simulink library "lib_BMS_2019b"  (R2020a)
settings: Solver=VariableStepAuto  StartTime=0.0  StopTime=10.0  RelTol=1e-3
undefined symbols (not defined in the file): OCVdata
libraries: simulink x4
settings Model: Creator=wzhao  LastModifiedBy="wei  zhao"
settings DebuggingCC: ArithmeticOperatorsInVariantConditions=warning
settings SFSimCC: CustomCodeUndefinedFunction=UseInterfaceOnly
settings RTWCC: GenCodeOnly=on

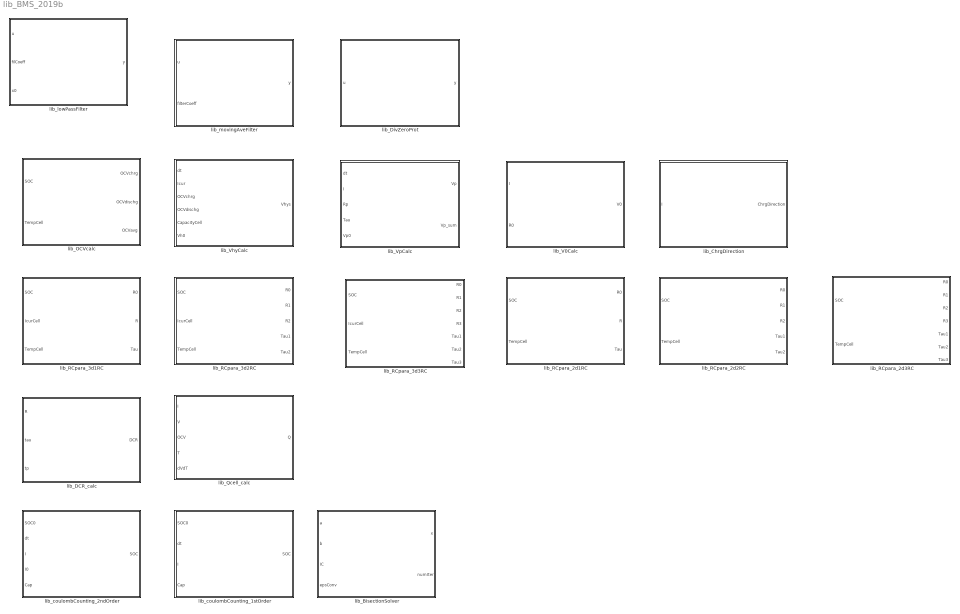
== system lib_BMS_2019b ==
  lib_BisectionSolver : Subsystem  TreatAsAtomicUnit=on  mask{myAlias_parameter=0, iterMax=10}
      mask prompts: myAlias_parameter "fx function data type"; iterMax "Maximum Iteration Number"
  lib_ChrgDirection : Subsystem  mask{ChrgFlag=0, DischrgFlag=0, Imin=0}
      mask prompts: ChrgFlag "Charge flag"; DischrgFlag "Discharge flag"; Imin "Min Current Tolerance"
  lib_DCR_calc : Subsystem  TreatAsAtomicUnit=on
  lib_DivZeroProt : Subsystem  TreatAsAtomicUnit=on  mask{epsilon=0, Default_value=0}
      mask prompts: epsilon "Divde-by-zero tolerance"; Default_value "Default Value"
  lib_OCVcalc : Subsystem  mask{OCVdata=OCVdata}
      mask prompts: OCVdata "OCV data."
  lib_Qcell_calc : Subsystem  TreatAsAtomicUnit=on
  lib_RCpara_2d1RC : Subsystem  TreatAsAtomicUnit=on  mask{xTemp=[1 2], xsoc=[1 2], yR0=zeros(2,2), yR=zeros(2,2), yTau=zeros(2,2)}
      mask prompts: xTemp "Temperature breakpoints"; xsoc "SOC breakpoints"; yR0 "R0 data"; yR "R data"; yTau "Tau data"
      mask DialogControl Container7 Prompt: Breakpoints
      mask DialogControl Container9 Prompt: RC data
  lib_RCpara_2d2RC : Subsystem  TreatAsAtomicUnit=on  mask{xTemp=[1 2], xsoc=[1 2], yR0=zeros(2,2), yR1=zeros(2,2), yR2=zeros(2,2), yTau1=zeros(2,2), yTau2=zeros(2,2)}
      mask prompts: xTemp "Temperature breakpoints"; xsoc "SOC breakpoints"; yR0 "R0 data"; yR1 "R1 data"; yR2 "R2 data"; yTau1 "Tau1 data"; yTau2 "Tau2 data"
      mask DialogControl Container7 Prompt: Breakpoints
      mask DialogControl Container9 Prompt: RC data
  lib_RCpara_2d3RC : Subsystem  TreatAsAtomicUnit=on  mask{xTemp=[1 2], xsoc=[1 2], yR0=zeros(2,2), yR1=zeros(2,2), yR2=zeros(2,2), yR3=zeros(2,2), yTau1=zeros(2,2), yTau2=zeros(2,2), yTau3=zeros(2,2)}
      mask prompts: xTemp "Temperature breakpoints"; xsoc "SOC breakpoints"; yR0 "R0 data"; yR1 "R1 data"; yR2 "R2 data"; yR3 "R3 data"; yTau1 "Tau1 data"; yTau2 "Tau2 data"; yTau3 "Tau3 data"
      mask DialogControl Container7 Prompt: Breakpoints
      mask DialogControl Container9 Prompt: RC data
  lib_RCpara_3d1RC : Subsystem  TreatAsAtomicUnit=on  mask{xsoc=[1 2], xIcurCell=[1 2], xTemp=[1 2], yR0=0, yR=zeros(2,2,2), yTau=zeros(2,2,2)}
      mask prompts: xsoc "SOC breakpoints"; xIcurCell "Current breakpoints"; xTemp "Temperature breakpoints"; yR0 "R0 data"; yR "R data"; yTau "Tau data"
      mask DialogControl Container7 Prompt: Breakpoints
      mask DialogControl Container10 Prompt: Tab
      mask DialogControl Container9 Prompt: RC data
  lib_RCpara_3d2RC : Subsystem  TreatAsAtomicUnit=on  mask{xsoc=[1 2], xIcurCell=[1 2], xTemp=[1 2], yR0=zeros(2,2,2), yR1=zeros(2,2,2), yR2=zeros(2,2,2), yTau1=zeros(2,2,2), yTau2=zeros(2,2,2)}
      mask prompts: xsoc "SOC breakpoints"; xIcurCell "Current breakpoints"; xTemp "Temperature breakpoints"; yR0 "R0 data"; yR1 "R1 data"; yR2 "R2 data"; yTau1 "Tau1 data"; yTau2 "Tau2 data"
      mask DialogControl Container7 Prompt: Breakpoints
      mask DialogControl Container9 Prompt: RC data
  lib_RCpara_3d3RC : Subsystem  TreatAsAtomicUnit=on  mask{xsoc=[1 2], xIcurCell=[1 2], xTemp=[1 2], yR0=zeros(2,2,2), yR1=zeros(2,2,2), yR2=zeros(2,2,2), yR3=zeros(2,2,2), yTau1=zeros(2,2,2), yTau2=zeros(2,2,2), yTau3=zeros(2,2,2)}
      mask prompts: xsoc "SOC breakpoints"; xIcurCell "Current breakpoints"; xTemp "Temperature breakpoints"; yR0 "R0 data"; yR1 "R1 data"; yR2 "R2 data"; yR3 "R3 data"; yTau1 "Tau1 data"; yTau2 "Tau2 data"; yTau3 "Tau3 data"
      mask DialogControl Container7 Prompt: Breakpoints
      mask DialogControl Container9 Prompt: RC data
  lib_V0Calc : Subsystem  TreatAsAtomicUnit=on
  lib_VhyCalc : Subsystem  mask{Isign=1, Vh_para=0}
      mask prompts: Isign "Current Sign Convention(+is charge, - is negative)"; Vh_para "Vh parameter"
  lib_VpCalc : Subsystem  TreatAsAtomicUnit=on
  lib_coulombCounting_1stOrder : Subsystem  mask{Isign=0, unitConv=0}
      mask prompts: Isign "Discharge Current Sign"; unitConv "Unit Conversion Factor"
  lib_coulombCounting_2ndOrder : Subsystem  mask{Isign=0, unitConv=0}
      mask prompts: Isign "Charge Current Sign"; unitConv "Unit Conversion factor"
  lib_lowPassFilter : Subsystem  TreatAsAtomicUnit=on  RTWFcnName=lib_lowPassFilter
  lib_movingAveFilter : Subsystem  TreatAsAtomicUnit=on  mask{x0=0}
      mask prompts: x0 "Initial filter states"

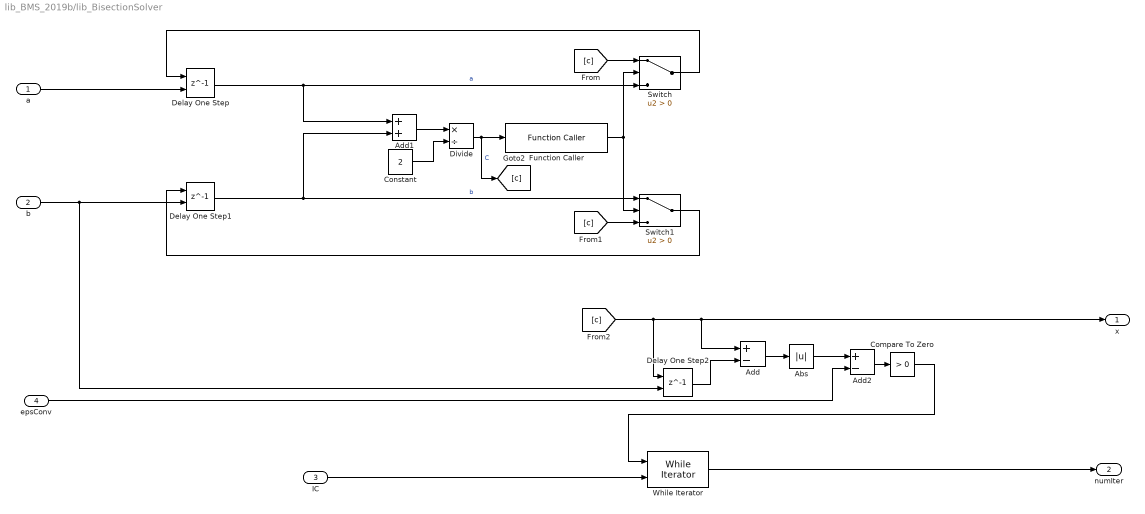
== system lib_BMS_2019b/lib_BisectionSolver ==
  a : Inport
  b : Inport  Port=2
  IC : Inport  Port=3
  epsConv : Inport  Port=4
  Abs : Abs
  Add : Sum  Inputs=+-
  Add1 : Sum
  Add2 : Sum  Inputs=+-
  Compare To Zero : simulink/Logic and Bit Operations/Compare To Zero  relop=>  OutDataTypeStr=boolean
  Constant : Constant  Value=2  OutDataTypeStr=Inherit: Inherit via back propagation  SampleTime=-1
  Delay One Step : Delay  DelayLength=1  InitialConditionSource=Input port
      settings: InputPortMap=u0,p4
  Delay One Step1 : Delay  DelayLength=1  InitialConditionSource=Input port
      settings: InputPortMap=u0,p4
  Delay One Step2 : Delay  DelayLength=1  InitialConditionSource=Input port
      settings: InputPortMap=u0,p4
  Divide : Product  Inputs=*/
  Function Caller : FunctionCaller  FunctionPrototype=y = funcToSolveBisec(u)  InputArgumentSpecifications=myAlias_parameter  OutputArgumentSpecifications=myAlias_parameter
  Switch : Switch  Criteria=u2 > Threshold
  Switch1 : Switch  Criteria=u2 > Threshold
  While Iterator : WhileIterator  MaxIters=iterMax  ResetStates=reset  ShowIterationPort=on
  x : Outport
  numIter : Outport  Port=2
  wires:
  IC/1 -> While Iterator/2
  [c] -> Add/1, x/1, Delay One Step2/1
  Delay One Step2/1 -> Add/2
  Add/1 -> Abs/1
  Abs/1 -> Add2/1
  Compare To Zero/1 -> While Iterator/1
  a/1 -> Delay One Step/2
  b/1 -> Delay One Step2/2, Delay One Step1/2
  Delay One Step/1 -> Add1/1, Switch/3  "a"
  Delay One Step1/1 -> Add1/2, Switch1/1  "b"
  Add1/1 -> Divide/1
  Constant/1 -> Divide/2
  Divide/1 -> [c], Function Caller/1  "C"
  Function Caller/1 -> Switch1/2, Switch/2
  [c] -> Switch/1
  [c] -> Switch1/3
  Switch/1 -> Delay One Step/1
  Switch1/1 -> Delay One Step1/1
  epsConv/1 -> Add2/2
  Add2/1 -> Compare To Zero/1
  While Iterator/1 -> numIter/1

== system lib_BMS_2019b/lib_ChrgDirection ==
  I : Inport
  Compare To Constant : simulink/Logic and Bit Operations/Compare To Constant  relop=>=  const=Imin  OutDataTypeStr=boolean
  Compare To Constant1 : simulink/Logic and Bit Operations/Compare To Constant  relop=<=  const=-Imin  OutDataTypeStr=boolean
  Constant : Constant  Value=ChrgFlag
  Constant1 : Constant  Value=DischrgFlag
  Switch : Switch  Criteria=u2 ~= 0
  Switch1 : Switch  Criteria=u2 ~= 0
  Unit Delay : UnitDelay  InitialCondition=ChrgFlag  SampleTime=-1  HasFrameUpgradeWarning=on
  ChrgDirection : Outport
  wires:
  I/1 -> Compare To Constant1/1, Compare To Constant/1
  Compare To Constant/1 -> Switch/2
  Constant/1 -> Switch/1
  Compare To Constant1/1 -> Switch1/2
  Switch1/1 -> Switch/3
  Constant1/1 -> Switch1/1
  Switch/1 -> ChrgDirection/1, Unit Delay/1
  Unit Delay/1 -> Switch1/3

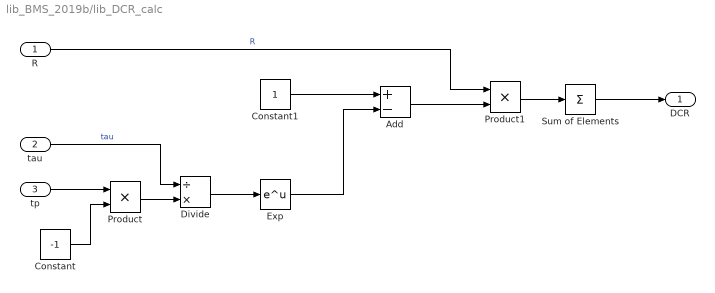
== system lib_BMS_2019b/lib_DCR_calc ==
  R : Inport
  tau : Inport  Port=2
  tp : Inport  Port=3
  Add : Sum  Inputs=+-
  Constant : Constant  Value=-1  OutDataTypeStr=Inherit: Inherit via back propagation
  Constant1 : Constant  OutDataTypeStr=Inherit: Inherit via back propagation
  Divide : Product  Inputs=/*
  Exp : Math  SaturateOnIntegerOverflow=on
  Product : Product
  Product1 : Product
  Sum of Elements : Sum  Inputs=+
  DCR : Outport
  wires:
  Sum of Elements/1 -> DCR/1
  tp/1 -> Product/1
  Constant/1 -> Product/2
  Product/1 -> Divide/2
  tau/1 -> Divide/1  "tau"
  Divide/1 -> Exp/1
  Exp/1 -> Add/2
  Product1/1 -> Sum of Elements/1
  Constant1/1 -> Add/1
  Add/1 -> Product1/2
  R/1 -> Product1/1  "R"

== system lib_BMS_2019b/lib_DivZeroProt ==
  u : Inport
  Abs : Abs
  Compare To Constant : simulink/Logic and Bit Operations/Compare To Constant  relop=<=  const=epsilon  OutDataTypeStr=boolean
  Constant2 : Constant  Value=Default_value
  Switch : Switch  Criteria=u2 ~= 0
  y : Outport
  wires:
  Constant2/1 -> Switch/1
  Compare To Constant/1 -> Switch/2
  u/1 -> Switch/3, Abs/1
  Abs/1 -> Compare To Constant/1
  Switch/1 -> y/1

== system lib_BMS_2019b/lib_OCVcalc ==
  SOC : Inport
  TempCell : Inport  Port=2
  1-D Lookup Table : Lookup_n-D  BreakpointsForDimension1=OCVdata.xSOC  BreakpointsForDimension2=OCVdata.xTemp  Table=OCVdata.yOCVc  InternalRulePriority=Speed  RndMeth=Simplest  InputSameDT=on
  1-D Lookup Table1 : Lookup_n-D  BreakpointsForDimension1=OCVdata.xSOC  BreakpointsForDimension2=OCVdata.xTemp  Table=OCVdata.yOCVd  InternalRulePriority=Speed  RndMeth=Simplest  InputSameDT=on
  Add : Sum
  Constant : Constant  Value=2  OutDataTypeStr=Inherit: Inherit via back propagation
  Divide : Product  Inputs=*/
  OCVchrg : Outport
  OCVdischg : Outport  Port=2
  OCVavg : Outport  Port=3
  wires:
  SOC/1 -> 1-D Lookup Table1/1, 1-D Lookup Table/1
  TempCell/1 -> 1-D Lookup Table1/2, 1-D Lookup Table/2
  1-D Lookup Table/1 -> Add/1, OCVchrg/1
  1-D Lookup Table1/1 -> OCVdischg/1, Add/2
  Add/1 -> Divide/1
  Constant/1 -> Divide/2
  Divide/1 -> OCVavg/1

== system lib_BMS_2019b/lib_Qcell_calc ==
  I : Inport
  V : Inport  Port=2
  OCV : Inport  Port=3
  T : Inport  Port=4
  dVdT : Inport  Port=5
  Abs : Abs
  Add : Sum  Inputs=-+
  Add1 : Sum
  Product : Product
  Product1 : Product  Inputs=3
  Q : Outport
  wires:
  V/1 -> Add/1
  OCV/1 -> Add/2
  Add/1 -> Product/2
  I/1 -> Product1/1, Product/1
  Product/1 -> Abs/1
  T/1 -> Product1/2
  dVdT/1 -> Product1/3
  Abs/1 -> Add1/1  "Qire"
  Product1/1 -> Add1/2  "Qrev"
  Add1/1 -> Q/1

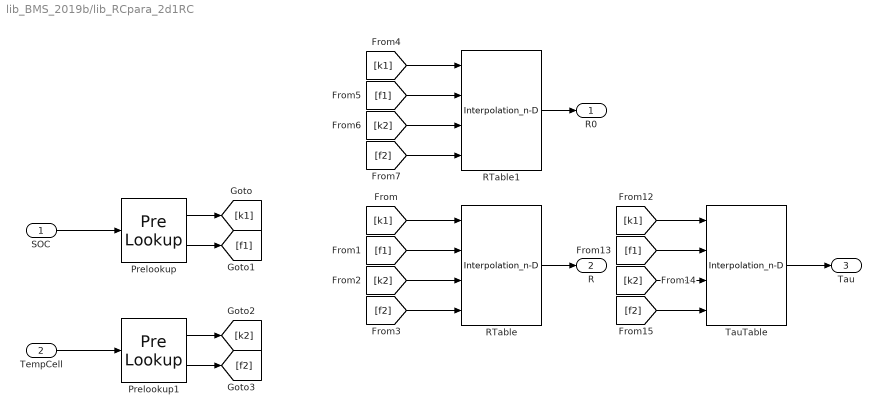
== system lib_BMS_2019b/lib_RCpara_2d1RC ==
  SOC : Inport
  TempCell : Inport  Port=2
  Prelookup : PreLookup  BreakpointsData=xsoc  ExtrapMethod=Linear
  Prelookup1 : PreLookup  BreakpointsData=xTemp  ExtrapMethod=Linear
  RTable : Interpolation_n-D  Table=yR  InternalRulePriority=Speed
  RTable1 : Interpolation_n-D  Table=yR0  InternalRulePriority=Speed
  TauTable : Interpolation_n-D  Table=yTau  InternalRulePriority=Speed
  R0 : Outport
  R : Outport  Port=2
  Tau : Outport  Port=3
  wires:
  Prelookup1/2 -> [f2]
  [k1] -> TauTable/1
  [f2] -> TauTable/4
  Prelookup/2 -> [f1]
  TauTable/1 -> Tau/1
  [k2] -> RTable/3
  [f2] -> RTable/4
  [k2] -> TauTable/3
  [f1] -> TauTable/2
  TempCell/1 -> Prelookup1/1
  Prelookup/1 -> [k1]
  [k1] -> RTable/1
  SOC/1 -> Prelookup/1
  Prelookup1/1 -> [k2]
  RTable/1 -> R/1
  [f1] -> RTable/2
  [f2] -> RTable1/4
  [f1] -> RTable1/2
  [k2] -> RTable1/3
  [k1] -> RTable1/1
  RTable1/1 -> R0/1

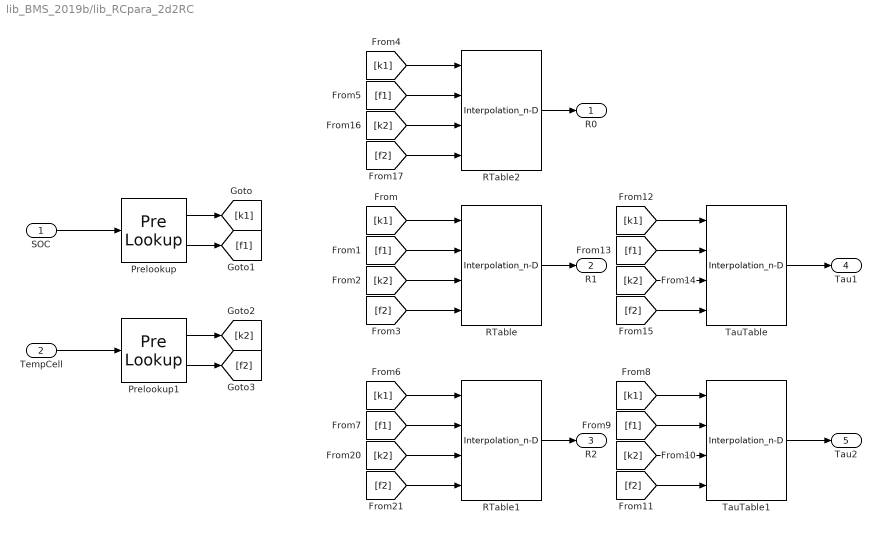
== system lib_BMS_2019b/lib_RCpara_2d2RC ==
  SOC : Inport
  TempCell : Inport  Port=2
  Prelookup : PreLookup  BreakpointsData=xsoc  ExtrapMethod=Linear
  Prelookup1 : PreLookup  BreakpointsData=xTemp  ExtrapMethod=Linear
  RTable : Interpolation_n-D  Table=yR1  InternalRulePriority=Speed
  RTable1 : Interpolation_n-D  Table=yR2  InternalRulePriority=Speed
  RTable2 : Interpolation_n-D  Table=yR0  InternalRulePriority=Speed
  TauTable : Interpolation_n-D  Table=yTau1  InternalRulePriority=Speed
  TauTable1 : Interpolation_n-D  Table=yTau2  InternalRulePriority=Speed
  R0 : Outport
  R1 : Outport  Port=2
  R2 : Outport  Port=3
  Tau1 : Outport  Port=4
  Tau2 : Outport  Port=5
  wires:
  Prelookup1/2 -> [f2]
  [k1] -> TauTable/1
  [f2] -> TauTable/4
  Prelookup/2 -> [f1]
  TauTable/1 -> Tau1/1
  [k2] -> RTable/3
  [f2] -> RTable/4
  [k2] -> TauTable/3
  [f1] -> TauTable/2
  TempCell/1 -> Prelookup1/1
  Prelookup/1 -> [k1]
  [k1] -> RTable/1
  SOC/1 -> Prelookup/1
  Prelookup1/1 -> [k2]
  RTable/1 -> R1/1
  [f1] -> RTable/2
  [f1] -> RTable1/2
  [k1] -> RTable1/1
  RTable1/1 -> R2/1
  [f2] -> RTable1/4
  [k2] -> TauTable1/3
  TauTable1/1 -> Tau2/1
  [k2] -> RTable1/3
  [f1] -> TauTable1/2
  [k1] -> TauTable1/1
  [f2] -> TauTable1/4
  [k1] -> RTable2/1
  [f1] -> RTable2/2
  [k2] -> RTable2/3
  [f2] -> RTable2/4
  RTable2/1 -> R0/1

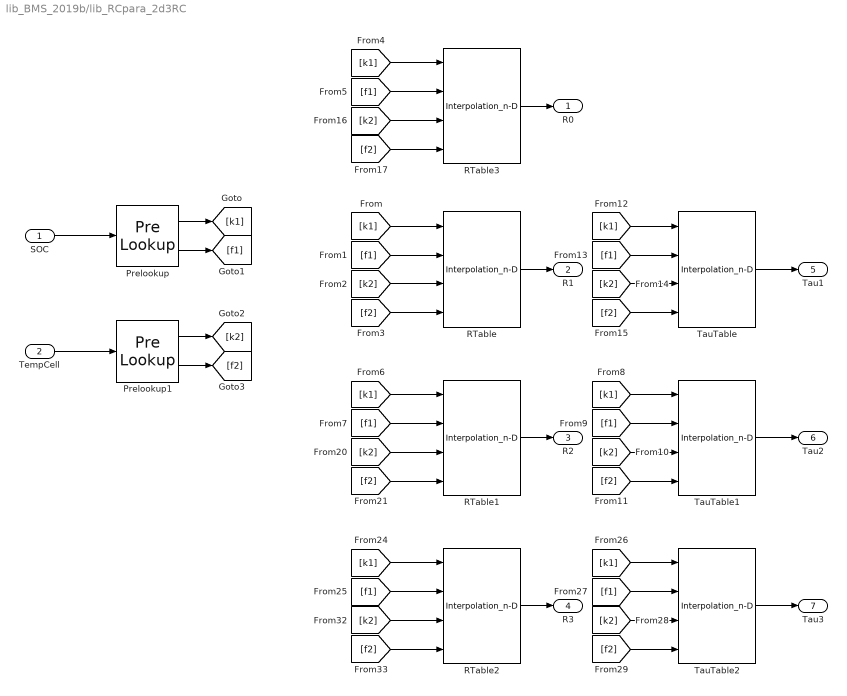
== system lib_BMS_2019b/lib_RCpara_2d3RC ==
  SOC : Inport
  TempCell : Inport  Port=2
  Prelookup : PreLookup  BreakpointsData=xsoc  ExtrapMethod=Linear
  Prelookup1 : PreLookup  BreakpointsData=xTemp  ExtrapMethod=Linear
  RTable : Interpolation_n-D  Table=yR1  InternalRulePriority=Speed
  RTable1 : Interpolation_n-D  Table=yR2  InternalRulePriority=Speed
  RTable2 : Interpolation_n-D  Table=yR3  InternalRulePriority=Speed
  RTable3 : Interpolation_n-D  Table=yR0  InternalRulePriority=Speed
  TauTable : Interpolation_n-D  Table=yTau1  InternalRulePriority=Speed
  TauTable1 : Interpolation_n-D  Table=yTau2  InternalRulePriority=Speed
  TauTable2 : Interpolation_n-D  Table=yTau3  InternalRulePriority=Speed
  R0 : Outport
  R1 : Outport  Port=2
  R2 : Outport  Port=3
  R3 : Outport  Port=4
  Tau1 : Outport  Port=5
  Tau2 : Outport  Port=6
  Tau3 : Outport  Port=7
  wires:
  Prelookup1/2 -> [f2]
  [k1] -> TauTable/1
  [f2] -> TauTable/4
  Prelookup/2 -> [f1]
  TauTable/1 -> Tau1/1
  [k2] -> RTable/3
  [f2] -> RTable/4
  [k2] -> TauTable/3
  [f1] -> TauTable/2
  TempCell/1 -> Prelookup1/1
  Prelookup/1 -> [k1]
  [k1] -> RTable/1
  SOC/1 -> Prelookup/1
  Prelookup1/1 -> [k2]
  RTable/1 -> R1/1
  [f1] -> RTable/2
  [f1] -> RTable1/2
  [k1] -> RTable1/1
  RTable1/1 -> R2/1
  [f2] -> RTable1/4
  [k2] -> TauTable1/3
  TauTable1/1 -> Tau2/1
  [k2] -> RTable1/3
  [f1] -> TauTable1/2
  [k1] -> TauTable1/1
  [f2] -> TauTable1/4
  [f1] -> RTable2/2
  [k1] -> RTable2/1
  RTable2/1 -> R3/1
  [f2] -> RTable2/4
  [k2] -> TauTable2/3
  TauTable2/1 -> Tau3/1
  [k2] -> RTable2/3
  [f1] -> TauTable2/2
  [k1] -> TauTable2/1
  [f2] -> TauTable2/4
  [f2] -> RTable3/4
  RTable3/1 -> R0/1
  [k1] -> RTable3/1
  [k2] -> RTable3/3
  [f1] -> RTable3/2

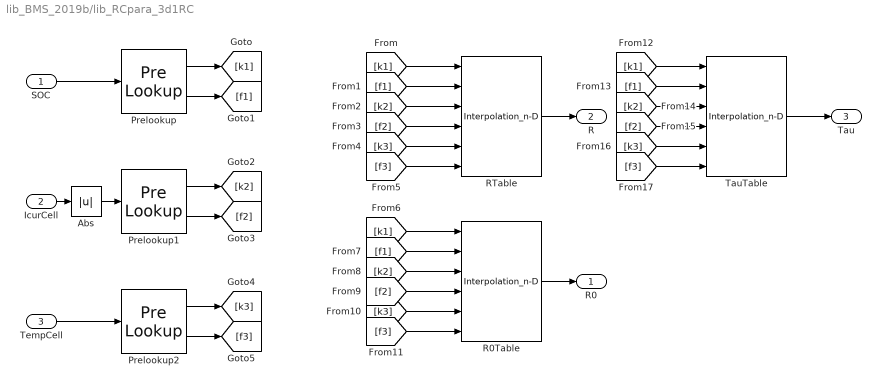
== system lib_BMS_2019b/lib_RCpara_3d1RC ==
  SOC : Inport
  IcurCell : Inport  Port=2
  TempCell : Inport  Port=3
  Abs : Abs
  Prelookup : PreLookup  BreakpointsData=xsoc  ExtrapMethod=Linear
  Prelookup1 : PreLookup  BreakpointsData=xIcurCell  ExtrapMethod=Linear
  Prelookup2 : PreLookup  BreakpointsData=xTemp  ExtrapMethod=Linear
  R0Table : Interpolation_n-D  NumberOfTableDimensions=3  Table=yR0  InternalRulePriority=Speed
      settings: InputPortMap=u0,u1,u2,u3,u4,u5
  RTable : Interpolation_n-D  NumberOfTableDimensions=3  Table=yR  InternalRulePriority=Speed
      settings: InputPortMap=u0,u1,u2,u3,u4,u5
  TauTable : Interpolation_n-D  NumberOfTableDimensions=3  Table=yTau  InternalRulePriority=Speed
      settings: InputPortMap=u0,u1,u2,u3,u4,u5
  R0 : Outport
  R : Outport  Port=2
  Tau : Outport  Port=3
  wires:
  Prelookup1/2 -> [f2]
  [k1] -> TauTable/1
  [f2] -> TauTable/4
  [k3] -> RTable/5
  Prelookup/2 -> [f1]
  TauTable/1 -> Tau/1
  [k2] -> RTable/3
  [f3] -> RTable/6
  [f2] -> RTable/4
  [f3] -> TauTable/6
  [k2] -> TauTable/3
  [k3] -> TauTable/5
  [f1] -> TauTable/2
  Prelookup/1 -> [k1]
  [k1] -> RTable/1
  SOC/1 -> Prelookup/1
  TempCell/1 -> Prelookup2/1
  Prelookup2/2 -> [f3]
  Prelookup2/1 -> [k3]
  Prelookup1/1 -> [k2]
  RTable/1 -> R/1
  [f1] -> RTable/2
  [k2] -> R0Table/3
  [f3] -> R0Table/6
  [k1] -> R0Table/1
  [f2] -> R0Table/4
  R0Table/1 -> R0/1
  [f1] -> R0Table/2
  [k3] -> R0Table/5
  IcurCell/1 -> Abs/1
  Abs/1 -> Prelookup1/1

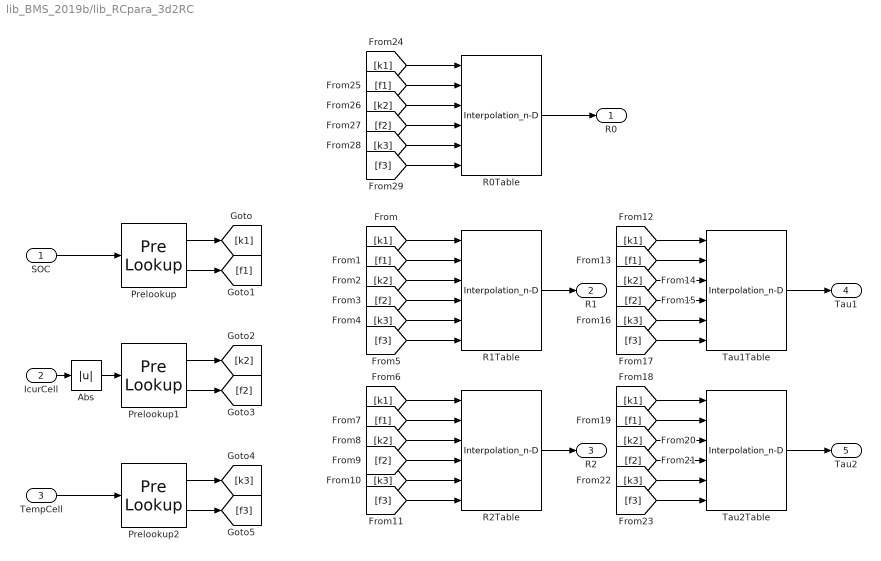
== system lib_BMS_2019b/lib_RCpara_3d2RC ==
  SOC : Inport
  IcurCell : Inport  Port=2
  TempCell : Inport  Port=3
  Abs : Abs
  Prelookup : PreLookup  BreakpointsData=xsoc  ExtrapMethod=Linear
  Prelookup1 : PreLookup  BreakpointsData=xIcurCell  ExtrapMethod=Linear
  Prelookup2 : PreLookup  BreakpointsData=xTemp  ExtrapMethod=Linear
  R0Table : Interpolation_n-D  NumberOfTableDimensions=3  Table=yR0  InternalRulePriority=Speed
      settings: InputPortMap=u0,u1,u2,u3,u4,u5
  R1Table : Interpolation_n-D  NumberOfTableDimensions=3  Table=yR1  InternalRulePriority=Speed
      settings: InputPortMap=u0,u1,u2,u3,u4,u5
  R2Table : Interpolation_n-D  NumberOfTableDimensions=3  Table=yR2  InternalRulePriority=Speed
      settings: InputPortMap=u0,u1,u2,u3,u4,u5
  Tau1Table : Interpolation_n-D  NumberOfTableDimensions=3  Table=yTau1  InternalRulePriority=Speed
      settings: InputPortMap=u0,u1,u2,u3,u4,u5
  Tau2Table : Interpolation_n-D  NumberOfTableDimensions=3  Table=yTau2  InternalRulePriority=Speed
      settings: InputPortMap=u0,u1,u2,u3,u4,u5
  R0 : Outport
  R1 : Outport  Port=2
  R2 : Outport  Port=3
  Tau1 : Outport  Port=4
  Tau2 : Outport  Port=5
  wires:
  Prelookup1/2 -> [f2]
  [k3] -> Tau2Table/5
  [k1] -> Tau1Table/1
  [f2] -> Tau1Table/4
  [k3] -> R1Table/5
  [f2] -> R2Table/4
  Prelookup/2 -> [f1]
  Tau1Table/1 -> Tau1/1
  [k2] -> R1Table/3
  [k1] -> R2Table/1
  [k1] -> Tau2Table/1
  [f3] -> R1Table/6
  R2Table/1 -> R2/1
  [f2] -> R1Table/4
  [f1] -> Tau2Table/2
  [f3] -> Tau1Table/6
  [k2] -> Tau1Table/3
  [k3] -> Tau1Table/5
  [f1] -> Tau1Table/2
  [k2] -> Tau2Table/3
  [f3] -> Tau2Table/6
  [f2] -> Tau2Table/4
  Prelookup/1 -> [k1]
  [k1] -> R1Table/1
  Tau2Table/1 -> Tau2/1
  SOC/1 -> Prelookup/1
  TempCell/1 -> Prelookup2/1
  Prelookup2/2 -> [f3]
  Prelookup2/1 -> [k3]
  Prelookup1/1 -> [k2]
  R1Table/1 -> R1/1
  [k3] -> R2Table/5
  [f1] -> R2Table/2
  [f1] -> R1Table/2
  [f3] -> R2Table/6
  [k2] -> R2Table/3
  [k2] -> R0Table/3
  [f3] -> R0Table/6
  [k3] -> R0Table/5
  [k1] -> R0Table/1
  [f1] -> R0Table/2
  [f2] -> R0Table/4
  R0Table/1 -> R0/1
  IcurCell/1 -> Abs/1
  Abs/1 -> Prelookup1/1

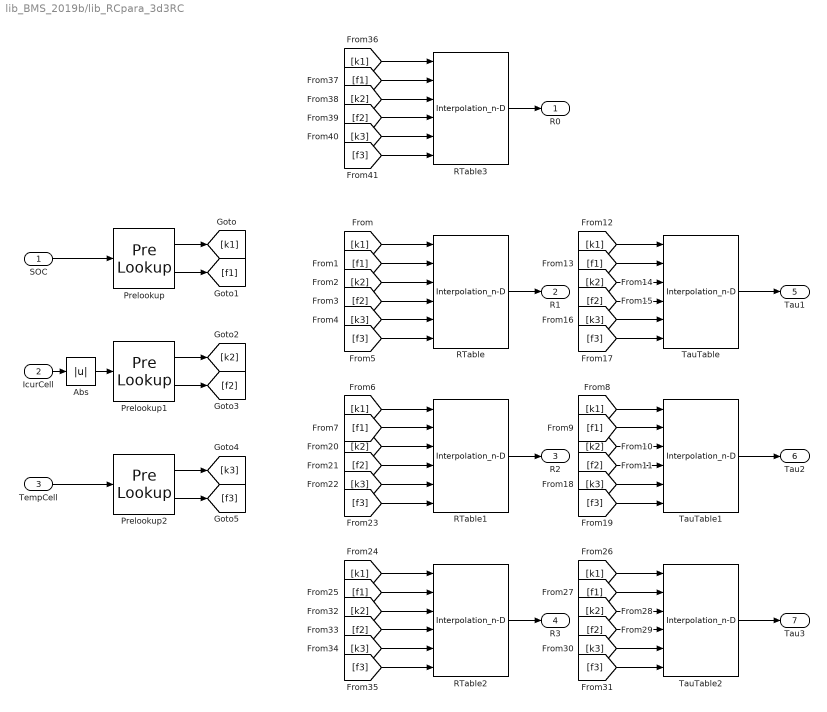
== system lib_BMS_2019b/lib_RCpara_3d3RC ==
  SOC : Inport
  IcurCell : Inport  Port=2
  TempCell : Inport  Port=3
  Abs : Abs
  Prelookup : PreLookup  BreakpointsData=xsoc  ExtrapMethod=Linear
  Prelookup1 : PreLookup  BreakpointsData=xIcurCell  ExtrapMethod=Linear
  Prelookup2 : PreLookup  BreakpointsData=xTemp  ExtrapMethod=Linear
  RTable : Interpolation_n-D  NumberOfTableDimensions=3  Table=yR1  InternalRulePriority=Speed
      settings: InputPortMap=u0,u1,u2,u3,u4,u5
  RTable1 : Interpolation_n-D  NumberOfTableDimensions=3  Table=yR2  InternalRulePriority=Speed
      settings: InputPortMap=u0,u1,u2,u3,u4,u5
  RTable2 : Interpolation_n-D  NumberOfTableDimensions=3  Table=yR3  InternalRulePriority=Speed
      settings: InputPortMap=u0,u1,u2,u3,u4,u5
  RTable3 : Interpolation_n-D  NumberOfTableDimensions=3  Table=yR0  InternalRulePriority=Speed
      settings: InputPortMap=u0,u1,u2,u3,u4,u5
  TauTable : Interpolation_n-D  NumberOfTableDimensions=3  Table=yTau1  InternalRulePriority=Speed
      settings: InputPortMap=u0,u1,u2,u3,u4,u5
  TauTable1 : Interpolation_n-D  NumberOfTableDimensions=3  Table=yTau2  InternalRulePriority=Speed
      settings: InputPortMap=u0,u1,u2,u3,u4,u5
  TauTable2 : Interpolation_n-D  NumberOfTableDimensions=3  Table=yTau3  InternalRulePriority=Speed
      settings: InputPortMap=u0,u1,u2,u3,u4,u5
  R0 : Outport
  R1 : Outport  Port=2
  R2 : Outport  Port=3
  R3 : Outport  Port=4
  Tau1 : Outport  Port=5
  Tau2 : Outport  Port=6
  Tau3 : Outport  Port=7
  wires:
  Prelookup1/2 -> [f2]
  [k1] -> TauTable/1
  [f2] -> TauTable/4
  [k3] -> RTable/5
  Prelookup/2 -> [f1]
  TauTable/1 -> Tau1/1
  [k2] -> RTable/3
  [f3] -> RTable/6
  [f2] -> RTable/4
  [f3] -> TauTable/6
  [k2] -> TauTable/3
  [k3] -> TauTable/5
  [f1] -> TauTable/2
  Prelookup/1 -> [k1]
  [k1] -> RTable/1
  SOC/1 -> Prelookup/1
  TempCell/1 -> Prelookup2/1
  Prelookup2/2 -> [f3]
  Prelookup2/1 -> [k3]
  Prelookup1/1 -> [k2]
  RTable/1 -> R1/1
  [f1] -> RTable/2
  [f1] -> RTable1/2
  [k1] -> RTable1/1
  RTable1/1 -> R2/1
  [f3] -> TauTable1/6
  [f3] -> RTable1/6
  [f2] -> RTable1/4
  [k2] -> TauTable1/3
  [k3] -> RTable1/5
  TauTable1/1 -> Tau2/1
  [k2] -> RTable1/3
  [f1] -> TauTable1/2
  [k1] -> TauTable1/1
  [f2] -> TauTable1/4
  [k3] -> TauTable1/5
  [f1] -> RTable2/2
  [k1] -> RTable2/1
  RTable2/1 -> R3/1
  [f3] -> TauTable2/6
  [f3] -> RTable2/6
  [f2] -> RTable2/4
  [k2] -> TauTable2/3
  [k3] -> RTable2/5
  TauTable2/1 -> Tau3/1
  [k2] -> RTable2/3
  [f1] -> TauTable2/2
  [k1] -> TauTable2/1
  [f2] -> TauTable2/4
  [k3] -> TauTable2/5
  IcurCell/1 -> Abs/1
  Abs/1 -> Prelookup1/1
  [k1] -> RTable3/1
  [f2] -> RTable3/4
  [k3] -> RTable3/5
  [f3] -> RTable3/6
  [k2] -> RTable3/3
  [f1] -> RTable3/2
  RTable3/1 -> R0/1

== system lib_BMS_2019b/lib_V0Calc ==
  I : Inport
  R0 : Inport  Port=2
  Product : Product
  V0 : Outport
  wires:
  I/1 -> Product/1
  R0/1 -> Product/2
  Product/1 -> V0/1

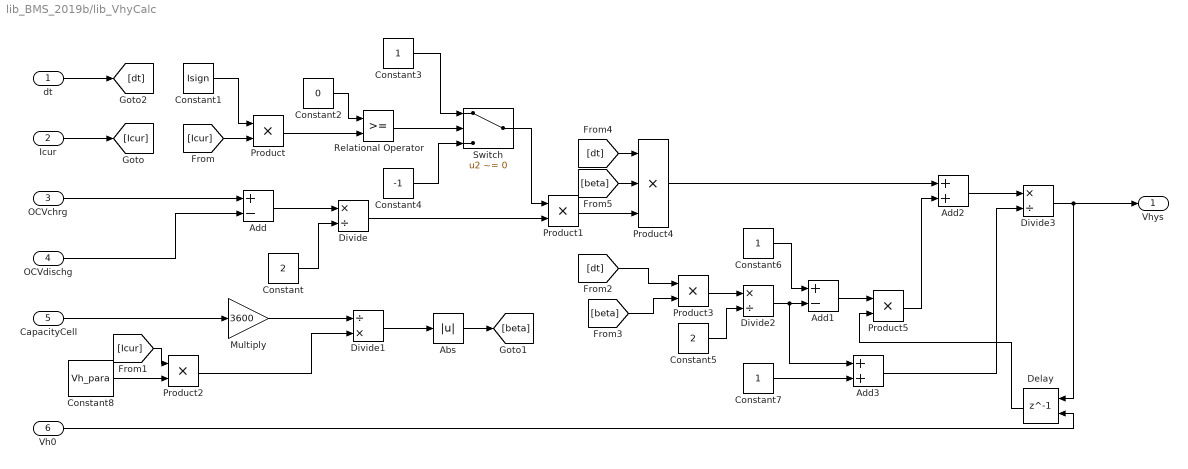
== system lib_BMS_2019b/lib_VhyCalc ==
  dt : Inport
  Icur : Inport  Port=2
  OCVchrg : Inport  Port=3
  OCVdischg : Inport  Port=4
  CapacityCell : Inport  Port=5
  Vh0 : Inport  Port=6
  Abs : Abs
  Add : Sum  Inputs=+-
  Add1 : Sum  Inputs=+-
  Add2 : Sum
  Add3 : Sum
  Constant : Constant  Value=2  OutDataTypeStr=Inherit: Inherit via back propagation
  Constant1 : Constant  Value=Isign  OutDataTypeStr=Inherit: Inherit via back propagation
  Constant2 : Constant  Value=0  OutDataTypeStr=Inherit: Inherit via back propagation
  Constant3 : Constant  OutDataTypeStr=Inherit: Inherit via back propagation
  Constant4 : Constant  Value=-1  OutDataTypeStr=Inherit: Inherit via back propagation
  Constant5 : Constant  Value=2  OutDataTypeStr=Inherit: Inherit via back propagation
  Constant6 : Constant  OutDataTypeStr=Inherit: Inherit via back propagation
  Constant7 : Constant  OutDataTypeStr=Inherit: Inherit via back propagation
  Constant8 : Constant  Value=Vh_para
  Delay : Delay  DelayLength=1  InitialConditionSource=Input port
      settings: InputPortMap=u0,p4
  Divide : Product  Inputs=*/
  Divide1 : Product  Inputs=/*
  Divide2 : Product  Inputs=*/
  Divide3 : Product  Inputs=*/
  Multiply : Gain  Gain=3600
  Product{,1..3,5} (5 alike) : Product
  Product4 : Product  Inputs=3
  Relational Operator : RelationalOperator  OutDataTypeStr=boolean  RndMeth=Simplest
  Switch : Switch  Criteria=u2 ~= 0
  Vhys : Outport
  wires:
  OCVchrg/1 -> Add/1
  OCVdischg/1 -> Add/2
  Add/1 -> Divide/1
  Constant/1 -> Divide/2
  Constant1/1 -> Product/1
  Product/1 -> Relational Operator/2
  Constant2/1 -> Relational Operator/1
  Relational Operator/1 -> Switch/2
  Constant3/1 -> Switch/1
  Constant4/1 -> Switch/3
  Switch/1 -> Product1/1
  Divide/1 -> Product1/2
  Icur/1 -> [Icur]
  [Icur] -> Product/2
  [Icur] -> Product2/1
  CapacityCell/1 -> Multiply/1
  Multiply/1 -> Divide1/1
  Product2/1 -> Divide1/2
  Divide1/1 -> Abs/1
  Abs/1 -> [beta]
  dt/1 -> [dt]
  [dt] -> Product3/1
  [beta] -> Product3/2
  Product3/1 -> Divide2/1
  Constant5/1 -> Divide2/2
  Divide2/1 -> Add3/1, Add1/2
  Constant6/1 -> Add1/1
  Product1/1 -> Product4/3
  [dt] -> Product4/1
  [beta] -> Product4/2
  Product4/1 -> Add2/1
  Add1/1 -> Product5/1
  Delay/1 -> Product5/2
  Product5/1 -> Add2/2
  Constant7/1 -> Add3/2
  Add2/1 -> Divide3/1
  Add3/1 -> Divide3/2
  Divide3/1 -> Vhys/1, Delay/1
  Vh0/1 -> Delay/2
  Constant8/1 -> Product2/2

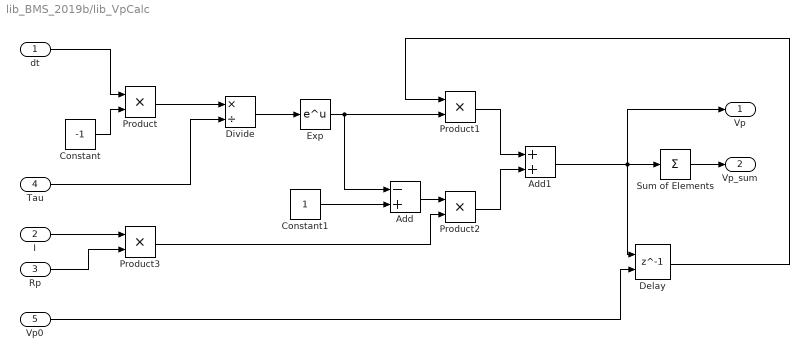
== system lib_BMS_2019b/lib_VpCalc ==
  dt : Inport
  I : Inport  Port=2
  Rp : Inport  Port=3
  Tau : Inport  Port=4
  Vp0 : Inport  Port=5
  Add : Sum  Inputs=-+
  Add1 : Sum
  Constant : Constant  Value=-1  OutDataTypeStr=Inherit: Inherit via back propagation
  Constant1 : Constant  OutDataTypeStr=Inherit: Inherit via back propagation
  Delay : Delay  DelayLength=1  InitialConditionSource=Input port
      settings: InputPortMap=u0,p4
  Divide : Product  Inputs=*/
  Exp : Math  SignedPower=on  SaturateOnIntegerOverflow=on
  Product{,1..3} (4 alike) : Product
  Sum of Elements : Sum  Inputs=+
  Vp : Outport
  Vp_sum : Outport  Port=2
  wires:
  Tau/1 -> Divide/2
  Delay/1 -> Product1/1
  Vp0/1 -> Delay/2
  Product2/1 -> Add1/2
  Product1/1 -> Add1/1
  Add/1 -> Product2/1
  Constant1/1 -> Add/2
  Exp/1 -> Product1/2, Add/1
  Add1/1 -> Sum of Elements/1, Vp/1, Delay/1
  Divide/1 -> Exp/1
  Constant/1 -> Product/2
  Product/1 -> Divide/1
  dt/1 -> Product/1
  Sum of Elements/1 -> Vp_sum/1
  I/1 -> Product3/1
  Rp/1 -> Product3/2
  Product3/1 -> Product2/2

== system lib_BMS_2019b/lib_coulombCounting_1stOrder ==
  SOC0 : Inport
  dt : Inport  Port=2
  I : Inport  Port=3
  Cap : Inport  Port=4
  Add1 : Sum
  Constant1 : Constant  Value=Isign  SampleTime=-1
  Constant2 : Constant  Value=unitConv  SampleTime=-1
  Divide1 : Product  Inputs=*/
  Product : Product
  Product1 : Product
  Product2 : Product
  SOC : Outport  VectorParamsAs1DForOutWhenUnconnected=off
  wires:
  Add1/1 -> SOC/1
  SOC0/1 -> Add1/1
  Product2/1 -> Add1/2
  Constant2/1 -> Product2/2
  Divide1/1 -> Product2/1
  Cap/1 -> Divide1/2
  Product1/1 -> Divide1/1
  dt/1 -> Product1/1
  Product/1 -> Product1/2
  Constant1/1 -> Product/2
  I/1 -> Product/1

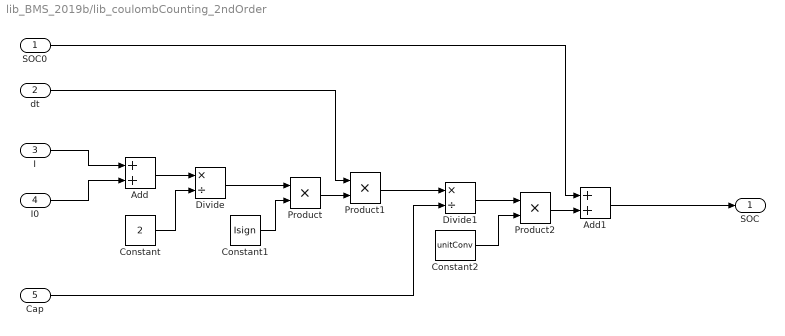
== system lib_BMS_2019b/lib_coulombCounting_2ndOrder ==
  SOC0 : Inport
  dt : Inport  Port=2
  I : Inport  Port=3
  I0 : Inport  Port=4
  Cap : Inport  Port=5
  Add : Sum
  Add1 : Sum
  Constant : Constant  Value=2  SampleTime=-1
  Constant1 : Constant  Value=Isign  SampleTime=-1
  Constant2 : Constant  Value=unitConv  SampleTime=-1
  Divide : Product  Inputs=*/
  Divide1 : Product  Inputs=*/
  Product : Product
  Product1 : Product
  Product2 : Product
  SOC : Outport  VectorParamsAs1DForOutWhenUnconnected=off
  wires:
  I/1 -> Add/1
  I0/1 -> Add/2
  Add/1 -> Divide/1
  Constant/1 -> Divide/2
  Divide/1 -> Product/1
  Constant1/1 -> Product/2
  Product/1 -> Product1/2
  dt/1 -> Product1/1
  Product1/1 -> Divide1/1
  Cap/1 -> Divide1/2
  Divide1/1 -> Product2/1
  Constant2/1 -> Product2/2
  Product2/1 -> Add1/2
  SOC0/1 -> Add1/1
  Add1/1 -> SOC/1

== system lib_BMS_2019b/lib_lowPassFilter ==
  u : Inport  OutDataTypeStr=single  PortDimensions=1
  filCoeff : Inport  Port=2  OutDataTypeStr=single  PortDimensions=1
  x0 : Inport  Port=3  OutDataTypeStr=single  PortDimensions=1
  Add : Sum  Inputs=-+
  Add1 : Sum
  Constant : Constant  OutDataTypeStr=Inherit: Inherit via back propagation
  Product : Product
  Product1 : Product
  y0 : Delay  DelayLength=1  InitialConditionSource=Input port
      settings: InputPortMap=u0,p4
  y : Outport  VectorParamsAs1DForOutWhenUnconnected=off
  wires:
  filCoeff/1 -> Add/1, Product/2
  Constant/1 -> Add/2
  Add/1 -> Product1/1
  u/1 -> Product1/2
  Product/1 -> Add1/1
  Product1/1 -> Add1/2
  Add1/1 -> y0/1, y/1
  y0/1 -> Product/1
  x0/1 -> y0/2

== system lib_BMS_2019b/lib_movingAveFilter ==
  u : Inport
  filterCoeff : Inport  Port=2
  Discrete FIR Filter : DiscreteFir  CoefSource=Input port  InitialStates=x0
      settings: InputPortMap=u0,u1
  y : Outport
  wires:
  u/1 -> Discrete FIR Filter/1
  Discrete FIR Filter/1 -> y/1
  filterCoeff/1 -> Discrete FIR Filter/2
